simulink model "CH"  (R2024a)
settings: Solver=VariableStepAuto  StartTime=0.0  StopTime=7000  FixedStep=1e-3  RelTol=1e-3
libraries: visionfilter x1, commrandsrc3 x1
(part 3 of 3)

== matlab function CH/MATLAB Function1 ==
  data: u input; y output
function y = PAM4_Mapping(u)
    
    out = 0;

    if(u == 0)
        out = -3;
    elseif(u == 1)
        out = -1;
    elseif(u == 2)
        out = 1;
    elseif(u == 3)
        out = 3;
    end
    
    y = out;
